simulink model "q2"  (R2020b)
settings: Solver=VariableStepAuto  StartTime=0.0  StopTime=10.0  RelTol=1e-3
values from neighbouring files (symbols this model uses):
  bp = .00005    (= 5e-05)    [q2_vars.m]
  br = 0.001    [q2_vars.m]
  g = 9.81    [q2_vars.m]
  Jp = mp*Lp*Lp/3    (= 0.000133128)    [q2_vars.m]
  Jr = mr*r*r/3    (= 0.000228791666667)    [q2_vars.m]
  Jt = Jr*Jp - (mp*r*l)^2    (= 1.31452806e-08)    [q2_vars.m]
  l = Lp/2    (= 0.0645)    [q2_vars.m]
  mp = 0.024    [q2_vars.m]
  r = 0.085    [q2_vars.m]
settings Model: Creator=Frienddo  LastModifiedBy=Frienddo

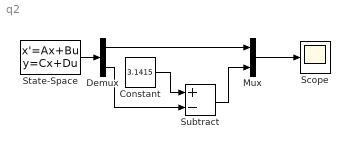
== system q2 ==
  Constant : Constant  Value=3.1415
  Demux : Demux  Outputs=2
  Mux : Mux  Inputs=2
  Scope : Scope
  State-Space : StateSpace  A=[0 1 0 0; 0 -Jp*br/Jt -((mp*l)^2)*r*g/Jt -mp*r*l*bp/Jt; 0 0 0 -1; 0 -mp*r*l*br/Jt -Jr*mp*g*l/Jt -Jr*bp/Jt]  B=[0; Jp/Jt; 0; mp*r*l/Jt]  C=[1 0 0 0; 0 0 1 0]  D=[0; 0]  InitialCondition=[0; 0; 3.1415-(3.1415+0.1); 0]
  Subtract : Sum  Inputs=+-
  wires:
  State-Space/1 -> Demux/1
  Demux/1 -> Mux/1
  Demux/2 -> Subtract/2
  Subtract/1 -> Mux/2
  Constant/1 -> Subtract/1
  Mux/1 -> Scope/1
